simulink model "model"  (R2013a)
settings: Solver=ode45  StartTime=0.0  StopTime=10.0  RelTol=1e-3
undefined symbols (not defined in the file): Hydride, Metal, Nickel
libraries: electricdrivelib x5, powerlib x1
settings Model: Creator=Simon  LastModifiedBy=Simon

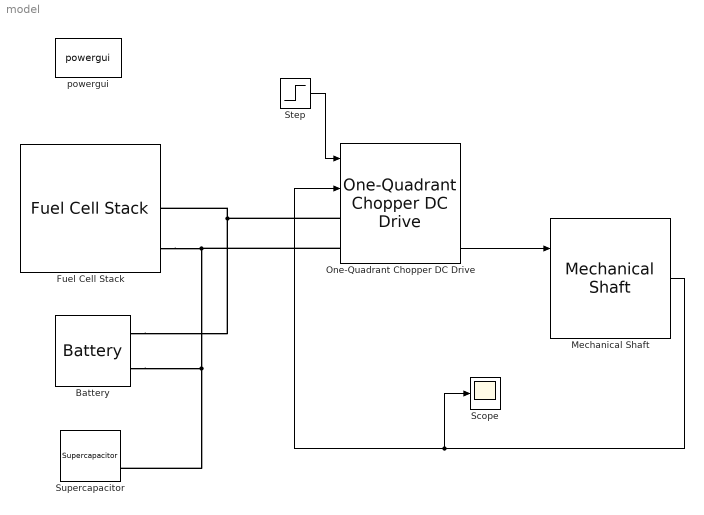
== system model ==
  Battery : electricdrivelib/Extra Sources/Battery  BatType=Nickel-Metal-Hydride  ShowDetailedParameters=off  NomV=42  NomQ=6.5  SOC=100  PresetModel=on  MaxQ=7  FullV=1.4136  Dis_rate=1.3  R=0.0018462  Normal_OP=6.25  expZone="[1.3017         1.3]"  Dis_Char=off  current=[6.5 13 32.5]  Units=Time  Batt_Tr=30
  Fuel Cell Stack : electricdrivelib/Extra Sources/Fuel Cell Stack  PresetModel=PEMFC - 1.26 kW - 24 Vdc  FcType=Proton Exchange Membrane (PEM)  Detailed=Detailed  Eoc="[42  35]"  NomVI="[52        24.23]"  EndVI="[100   20]"  Nc=42  n=46  TOp=55  AirFr=2400  SuppPress="[1.5           1]"  Comp="[99.95           21            1]"  plot_graph=off  ViewParam=off  SignX=off  SignY=off  FlowRateH2=off  FlowRateAir=off  SystemTemp=off  SystemPH2=off  SystemPAir=off  FCDyn=off  FC_tau=1  Peak_O2=80  V_Under=10
  Mechanical Shaft : electricdrivelib/Shafts and speed reducers/Mechanical Shaft  PresetModel=01 : Tln = 200 N-m  Ksh=17190  Bsh=600
  One-Quadrant Chopper DC Drive : electricdrivelib/DC drives/One-Quadrant Chopper DC Drive  showMaskWarnings=on  AverageValue=off  MechanicalLoad=Torque Tm  driveType=DC5
  Scope : Scope
      settings: YMin=-2e-05  YMax=3.75e-05
  Step : Step  Time=100  SampleTime=0
  Supercapacitor : electricdrivelib/Extra Sources/Supercapacitor  C=500  Rdc=2.1e-3  Voltage=16  Vmax=17  Ns=6  Np=1  Vinit=16  If=5.2e-3  PresetModel=off  Nc=6  r=1.23e-9  deltaV=0.3  alpha=0.3  Temp=25  demandeplot=off  I=10.2  sec=1988
  powergui : powerlib/powergui  Priority=1  SimulationMode=Discrete  SolverType=Tustin  SampleTime=1e-6  frequency=60  SPID=off  DisableSnubberDevices=off  DisableRonSwitches=off  DisableVfSwitches=off  SwTol=0  Interpol=off  DisplayEquations=off  frequencyindice=0  Pbase=100e6  ErrMax=1e-4  Iterations=50  UnitsV=kV  UnitsW=MW  FunctionMessages=off  echomessages=off  HookPort=off  EnableUseOfTLC=off  x0status=blocks  RestoreLinks=warning  ResistiveCurrentMeasurement=off  Frange=[0:2:500]  Ylog=off  Xlog=on  ShowGrid=off  save=off  variable=ZData  ZoomFFT=off  StartTime=0.0  cycles=1  DisplayStyle=1  fundamental=60  FreqAxis=off  MaxFrequency=1000  frequencyindicesteady=1  RmsSteady=1  display=off  Ts=0  methode=off
  wires:
  One-Quadrant Chopper DC Drive/4 -> Mechanical Shaft/1
  Mechanical Shaft/1 -> Scope/1, One-Quadrant Chopper DC Drive/2
  Step/1 -> One-Quadrant Chopper DC Drive/1
  connections:
  Fuel Cell Stack/RConn2 -- One-Quadrant Chopper DC Drive/LConn2 -- Battery/LConn2 -- Supercapacitor/LConn2
  One-Quadrant Chopper DC Drive/LConn1 -- Battery/LConn1 -- Fuel Cell Stack/RConn1
